simulink model "A_search_2021b"  (R2021b)
settings: Solver=ode1  StartTime=0.0  StopTime=inf  FixedStep=0.65  RelTol=1e-3
libraries: TcTargetLib x7
settings Model: Creator=ATLabor  LastModifiedBy=ATLabor
settings OptimizationCC: DefaultParameterBehavior=Inlined  LocalBlockOutputs=off  ZeroExternalMemoryAtStartup=off  ZeroInternalMemoryAtStartup=off
settings RTWCC: Description=TwinCAT GRT Target  SystemTargetFile=TwinCatGrt.tlc  GenCodeOnly=on  TemplateMakefile=tcgrt_msbuild.tmf  TargetLang=C++
settings STFCustomTargetCC: TargetLangStandard=C++11 (ISO)  CombineOutputUpdateFcns=on  CodeInterfacePackaging=C++ class  CPPClassGenCompliant=on  GRTInterface=off  SystemTargetFile=TwinCatGrt.tlc
settings GRTTargetCC: TargetLangStandard=C++11 (ISO)  ParMdlRefBuildCompliant=off  CompOptLevelCompliant=off  ConcurrentExecutionCompliant=off  MatFileLogging=off  CodeInterfacePackaging=C++ class  UseToolchainInfoCompliant=off  ExtModeMexFile=TcExtModeClient

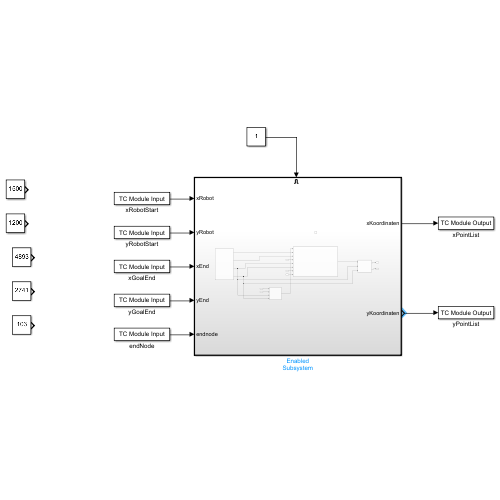
[thumbnail: Simulink's stored preview of the top-level diagram]
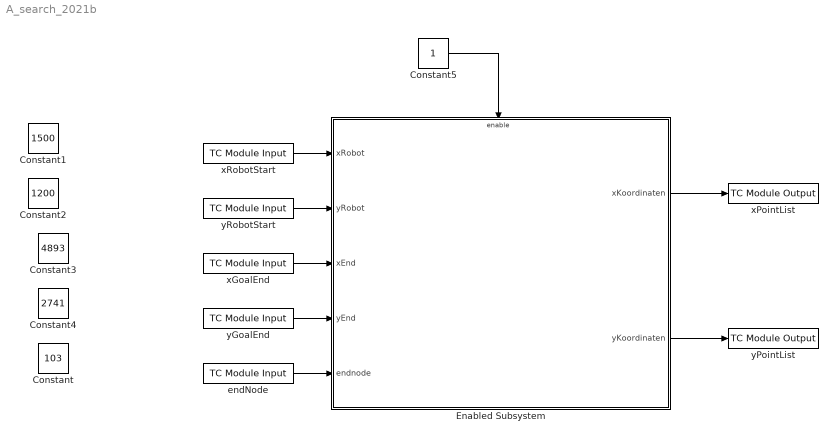
== system A_search_2021b ==
  Constant : Constant  Value=103
  Constant1 : Constant  Value=1500
  Constant2 : Constant  Value=1200
  Constant3 : Constant  Value=4893
  Constant4 : Constant  Value=2741
  Constant5 : Constant
  Enabled Subsystem : Subsystem  TreatAsAtomicUnit=on
  endNode : TcTargetLib/TC Module Input  PortDataType=double  PortDim=1  Value=0  SampleTime=-1  CodeGenConnectType=DataArea (InputDst)  DataTypeOverride=off
      settings: SourceProductName=Beckhoff TwinCAT Target
  xGoalEnd : TcTargetLib/TC Module Input  PortDataType=double  PortDim=1  Value=0  SampleTime=-1  CodeGenConnectType=DataArea (InputDst)  DataTypeOverride=off
      settings: SourceProductName=Beckhoff TwinCAT Target
  xPointList : TcTargetLib/TC Module Output  PortDataType=double  PortDim=144:1  SampleTime=-1  CodeGenConnectType=DataArea (OutputSrc)  DataTypeOverride=off
      settings: SourceProductName=Beckhoff TwinCAT Target
  xRobotStart : TcTargetLib/TC Module Input  PortDataType=double  PortDim=1  Value=0  SampleTime=-1  CodeGenConnectType=DataArea (InputDst)  DataTypeOverride=off
      settings: SourceProductName=Beckhoff TwinCAT Target
  yGoalEnd : TcTargetLib/TC Module Input  PortDataType=double  PortDim=1  Value=0  SampleTime=-1  CodeGenConnectType=DataArea (InputDst)  DataTypeOverride=off
      settings: SourceProductName=Beckhoff TwinCAT Target
  yPointList : TcTargetLib/TC Module Output  PortDataType=double  PortDim=144:1  SampleTime=-1  CodeGenConnectType=DataArea (OutputSrc)  DataTypeOverride=off
      settings: SourceProductName=Beckhoff TwinCAT Target
  yRobotStart : TcTargetLib/TC Module Input  PortDataType=double  PortDim=1  Value=0  SampleTime=-1  CodeGenConnectType=DataArea (InputDst)  DataTypeOverride=off
      settings: SourceProductName=Beckhoff TwinCAT Target
  wires:
  Enabled Subsystem/1(xKoordinaten) -> xPointList/1
  Enabled Subsystem/2(yKoordinaten) -> yPointList/1
  Constant5/1 -> Enabled Subsystem/Enable
  xRobotStart/1 -> Enabled Subsystem/1(xRobot)
  yRobotStart/1 -> Enabled Subsystem/2(yRobot)
  xGoalEnd/1 -> Enabled Subsystem/3(xEnd)
  yGoalEnd/1 -> Enabled Subsystem/4(yEnd)
  endNode/1 -> Enabled Subsystem/5(endnode)

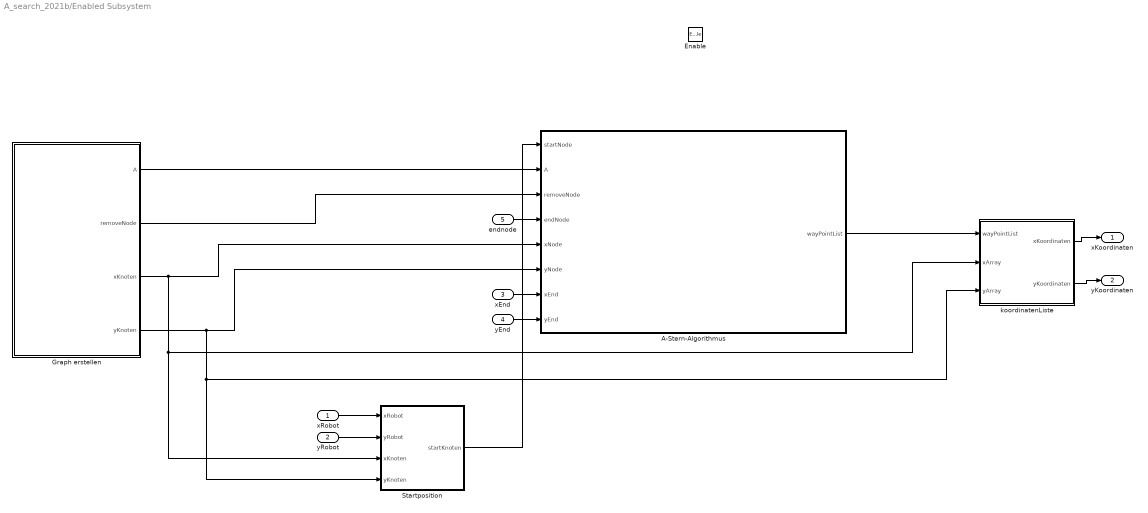
== system A_search_2021b/Enabled Subsystem ==
  xRobot : Inport
  yRobot : Inport  Port=2
  xEnd : Inport  Port=3
  yEnd : Inport  Port=4
  endnode : Inport  Port=5
  Enable : EnablePort
  A-Stern-Algorithmus : MATLAB Function  TreatAsAtomicUnit=on
  Graph erstellen : MATLAB Function  TreatAsAtomicUnit=on
  Startposition : MATLAB Function  TreatAsAtomicUnit=on
  koordinatenListe : MATLAB Function  TreatAsAtomicUnit=on
  xKoordinaten : Outport
  yKoordinaten : Outport  Port=2
  wires:
  koordinatenListe/1(xKoordinaten) -> xKoordinaten/1
  koordinatenListe/2(yKoordinaten) -> yKoordinaten/1
  Startposition/1(startKnoten) -> A-Stern-Algorithmus/1(startNode)
  A-Stern-Algorithmus/1(wayPointList) -> koordinatenListe/1(wayPointList)
  endnode/1 -> A-Stern-Algorithmus/4(endNode)
  xEnd/1 -> A-Stern-Algorithmus/7(xEnd)
  yEnd/1 -> A-Stern-Algorithmus/8(yEnd)
  xRobot/1 -> Startposition/1(xRobot)
  yRobot/1 -> Startposition/2(yRobot)
  Graph erstellen/1(A) -> A-Stern-Algorithmus/2(A)
  Graph erstellen/2(removeNode) -> A-Stern-Algorithmus/3(removeNode)
  Graph erstellen/3(xKnoten) -> koordinatenListe/2(xArray), Startposition/3(xKnoten), A-Stern-Algorithmus/5(xNode)
  Graph erstellen/4(yKnoten) -> Startposition/4(yKnoten), koordinatenListe/3(yArray), A-Stern-Algorithmus/6(yNode)

== matlab function A_search_2021b/Enabled Subsystem/Graph erstellen ==
  data: A output; removeNode output; xKnoten output; yKnoten output
function [A, removeNode, xKnoten, yKnoten]= fcn

numberOfNodes = 144;
numberOfColumns = 18;
A = zeros(numberOfNodes);

% Verbindung zu relevanten Knoten
for i = 1:numberOfNodes
    if i-1>0 && mod(i, numberOfColumns) ~= 1
        A(i-1,i) = 1000;
    end
    if i+1<numberOfNodes+1 && mod(i,numberOfColumns) ~= 0
        A(i+1,i)= 1000;
    end
    if i+numberOfColumns<numberOfNodes+1
        A(i+numberOfColumns,i)=1000;
    end
    if i-numberOfColumns>0
        A(i-numberOfColumns,i)=1000;
    end
    if i+numberOfColumns+1 < numberOfNodes+1 && mod(i,numberOfColumns) ~= 0
        A(i+numberOfColumns+1,i) = sqrt(2)*1000;
    end
    if i+numberOfColumns-1 < numberOfNodes+1 && mod(i, numberOfColumns) ~= 1
        A(i+numberOfColumns-1,i) = sqrt(2)*1000;
    end
     if i-numberOfColumns+1 > 0 && mod(i,numberOfColumns) ~= 1
        A(i-numberOfColumns+1,i) = sqrt(2)*1000;
    end
    if i-numberOfColumns-1 > 0 && mod(i, numberOfColumns) ~= 0
        A(i-numberOfColumns-1,i) = sqrt(2)*1000;
    end
end

% Lösen der Station
removeNode = [93 96 99 102 111 114 117 120 124 125 142 143];
for counter = 1:12
    for j = 1:numberOfNodes
        A(removeNode(counter),j) = 0;
        A(j,removeNode(counter)) = 0;
    end
end

% Umrechung von Knoten in Koordinaten
xKnoten = zeros(numberOfNodes,1);
yKnoten = zeros(numberOfNodes,1);
row = 600;
col = 200;
for i = 1:numberOfNodes
    xKnoten(i) = col;
    yKnoten(i) = row;
    col = col + 400;
    if mod(i,numberOfColumns) == 0 
        col = 200;
        row = row + 400;
    end 
end

== matlab function A_search_2021b/Enabled Subsystem/A-Stern-Algorithmus ==
  data: startNode input; wayPointList output; A input; removeNode input; endNode input; xNode input; yNode input; xEnd input; yEnd input
function wayPointList = fcn(startNode, A,removeNode, endNode, xNode, yNode, xEnd, yEnd)
numNodes = 144;
openList = zeros(8,5); %1. Node 2. g(x) 3. h(x) 4. f(x) 5. parent node
closedList = zeros(144,5); %1. Node 2. g(x) 3. h(x) 4. f(x) 5. parent node
neighborList = zeros(8,5); %1. Node 2. g(x) 3. h(x) 4. f(x) 5. parent node
step = 1;
index = 1;
overlap = false;
nodefmin = 0;
currentNode = startNode;
parentNode = 0;
noPath = false;
g = 0;
gprev = g;
h = sqrt(power(xNode(startNode)-xEnd,2) + power(yNode(startNode)-yEnd,2));
f = g + h;
fmin = 0;

%Goal reached?
while currentNode ~= endNode
    for counter = 1:14
        %The currentnode isn't a hinderance
        if currentNode ~= removeNode(counter)
            noHinderance = true;
        %The currentnode is a hinderance
        else
            noHinderance = false;
            break;
        end
    end
   if noHinderance == true 
        %The smallest f is put in closedlist when 
        closedList(step, 1) = currentNode;
        closedList(step, 2) = g;
        closedList(step, 3) = h;
        closedList(step, 4) = f;
        closedList(step, 5) = parentNode;
        step = step + 1;

        %Clear the openlist and neighborlist
        openList = zeros(8,5);
        neighborList = zeros(8,5);
        index = 1;
    
        %Search the neighbor and put in the neighborlist
        for i = 1:numNodes
            %calculate fowards
            if A(currentNode,i) ~= 0
                g = gprev + sqrt(power(xNode(i)-xNode(startNode),2) + power(yNode(i)-yNode(startNode),2));
                h = sqrt(power(xNode(i)-xEnd,2) + power(yNode(i)-yEnd,2));
                neighborList(index,1) = i;
                neighborList(index,2) = g;
                neighborList(index,3) = h;
                neighborList(index,4) = g + h;
                neighborList(index,5) = currentNode;
                index = index + 1;
            end
        end
    
        %the possible neighbors will be inserted in the openlist when it
        %doesn't exist in closedlist
        for i = 1:size(neighborList,1)
            for j = 1:size(closedList,1)
                if neighborList(i) == closedList(j)
                    overlap = true;
                    break;
                end
            end
            if overlap == false
                openList(i,1) = neighborList(i,1);
                openList(i,2) = neighborList(i,2);
                openList(i,3) = neighborList(i,3);
                openList(i,4) = neighborList(i,4);
                openList(i,5) = neighborList(i,5);
            end
            overlap = false;
        end
   else
       openList(nodefmin,:) = [];
   end

    %Search the smallest f in openlist
    flag = false; 
    for i = 1:size(openList,1)
        if openList(i,4) ~= 0
            if flag == false
                fmin = openList(i,4);
                nodefmin = i;
                flag = true;
            end
            if fmin > openList(i,4) 
                fmin = openList(i,4);
                nodefmin = i;
            end   
        end
    end

    %found the smallest f and update the values
    currentNode = openList(nodefmin,1);
    g = openList(nodefmin,2);
    h = openList(nodefmin,3);
    f = openList(nodefmin,4);
    parentNode = openList(nodefmin,5);
    gprev = g;
end

closedList(step, 1) = currentNode;
closedList(step, 2) = g;
closedList(step, 3) = h;
closedList(step, 4) = f;
closedList(step, 5) = parentNode;

wayPointList = zeros(144,1);
for index = 1:step
    wayPointList(index) = closedList(index,1);
end

== matlab function A_search_2021b/Enabled Subsystem/Startposition ==
  data: xRobot input; startKnoten output; yRobot input; xKnoten input; yKnoten input
function startKnoten= fcn(xRobot, yRobot, xKnoten, yKnoten)

startKnoten = 0;
startKnotenArray = 0;
diff_x = zeros(size(xKnoten,1),1);
diff_y = zeros(size(yKnoten,1),1);

for i = 1:size(xKnoten,1)
    diff_x(i) = abs(xRobot-xKnoten(i));
end

for i = 1:size(yKnoten,1)
    diff_y(i) = abs(yRobot-yKnoten(i));
end

xMin = min(diff_x);
yMin = min(diff_y);

xStart = find(diff_x == xMin);
yStart = find(diff_y == yMin);

startKnotenArray = intersect(xStart, yStart);

startKnoten = startKnotenArray(1,1);

== matlab function A_search_2021b/Enabled Subsystem/koordinatenListe ==
  data: wayPointList input; xKoordinaten output; yKoordinaten output; xArray input; yArray input
function [xKoordinaten, yKoordinaten]= fcn(wayPointList, xArray, yArray)

sizeList = size(wayPointList,1);
xKoordinaten = zeros(sizeList,1);
yKoordinaten = zeros(sizeList,1);

for i = 1 : sizeList
    if wayPointList ~= 0
        xKoordinaten(i) = xArray(wayPointList(i));
        yKoordinaten(i) = yArray(wayPointList(i));
    end
end
